simulink model "adaptiveControl_1DOF"  (R2021a)
settings: Solver=VariableStepAuto  StartTime=0.0  StopTime=50  RelTol=1e-3
values from neighbouring files (symbols this model uses):
  A = 0.2    [assignment8_main.m]
  Kd = 20    [assignment8_main.m]
  Khat_theta = 0.001    [assignment8_main.m]
  lambda = 10    [assignment8_main.m]
  omega = 0.5    [assignment8_main.m]
  theta_true = [myRobot_1DOF.I, myRobot_1DOF.F, myRobot_1DOF.G].'    [assignment8_main.m]
undefined symbols (not defined in the file or in its folder): myRobot_1DOF
settings Model: Creator=fabio  LastModifiedBy=fabio

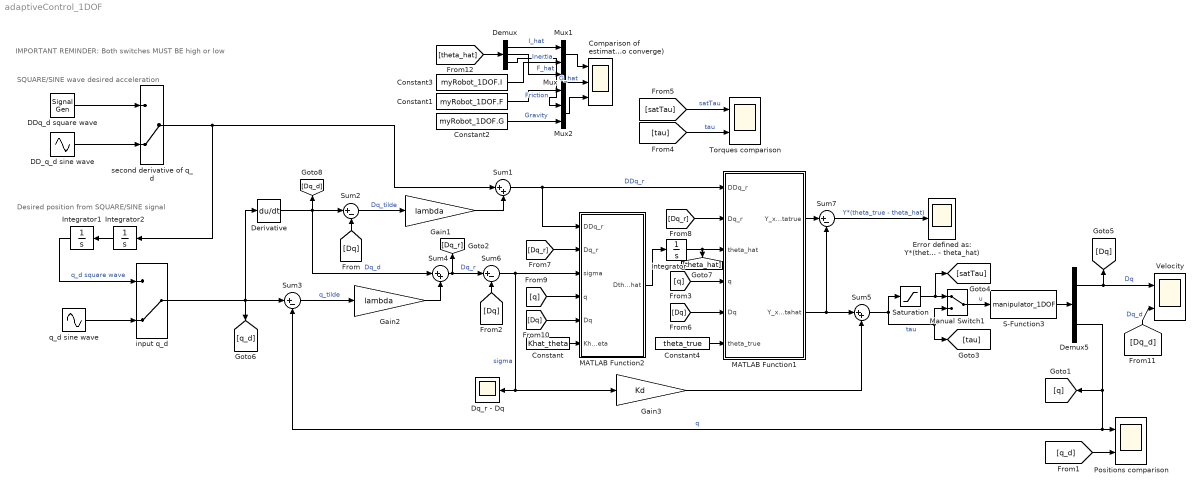
== system adaptiveControl_1DOF ==
  note: Desired position from SQUARE/SINE signal
  note: SQUARE/SINE wave desired acceleration
  note: IMPORTANT REMINDER: Both switches MUST BE high or low
  Comparison of estimated and real parameters (they don't necessarely have to converge) : Scope  NumInputPorts=3
  Constant : Constant  Value=Khat_theta  VectorParams1D=off
  Constant1 : Constant  Value=myRobot_1DOF.F
  Constant2 : Constant  Value=myRobot_1DOF.G
  Constant3 : Constant  Value=myRobot_1DOF.I  VectorParams1D=off
  Constant4 : Constant  Value=theta_true
  "DD_q_d sine wave " : Sin  Amplitude=-A*omega*omega  Frequency=omega  SampleTime=0
  DDq_d square wave : SignalGenerator  WaveForm=square  Amplitude=A  Frequency=omega*2  Units=rad/sec
  Demux : Demux  Outputs=3
  Demux5 : Demux  Outputs=[1 1]
  Derivative : Derivative
  Dq_r - Dq : Scope
  Error defined as: Y*(theta_true - theta_hat) : Scope
  Gain1 : Gain  Gain=lambda
  Gain2 : Gain  Gain=lambda
  Gain3 : Gain  Gain=Kd
  Integrator : Integrator  InitialCondition=myRobot_1DOF.theta_hat_0
  Integrator1 : Integrator
  Integrator2 : Integrator
  MATLAB Function1 : MATLAB Function  TreatAsAtomicUnit=on
  MATLAB Function2 : MATLAB Function  TreatAsAtomicUnit=on
  Manual Switch1 : ManualSwitch
  Mux : Mux  Inputs=2
  Mux1 : Mux  Inputs=2
  Mux2 : Mux  Inputs=2
  Positions comparison : Scope  NumInputPorts=2
  S-Function3 : S-Function  FunctionName=manipulator_1DOF  Parameters=myRobot_1DOF  SFunctionDeploymentMode=off  EnableBusSupport=off
  Saturation : Saturate  UpperLimit=20  LowerLimit=-20
  Sum1 : Sum  Inputs=|++
  Sum{2..3,6..7} (4 alike) : Sum  Inputs=|+-
  Sum4 : Sum  Inputs=|++
  Sum5 : Sum  Inputs=|++
  Torques comparison : Scope  NumInputPorts=2
  Velocity : Scope  NumInputPorts=2
  input q_d : ManualSwitch  CurrentSetting=0
  q_d sine wave : Sin  Amplitude=A  Frequency=omega  SampleTime=0
  second derivative of q_d : ManualSwitch  CurrentSetting=0
  wires:
  Manual Switch1/1 -> S-Function3/1  "u"
  Sum2/1 -> Gain1/1  "Dq_tilde"
  Saturation/1 -> Manual Switch1/1, [satTau]
  S-Function3/1 -> Demux5/1
  Demux5/1 -> [Dq], Velocity/1  "Dq"
  Demux5/2 -> Sum3/2, Positions comparison/1, [q]  "q"
  Sum3/1 -> Gain2/1  "q_tilde"
  Derivative/1 -> Sum4/1, Sum2/1, [Dq_d]  "Dq_d"
  Gain1/1 -> Sum1/2
  Gain2/1 -> Sum4/2
  Sum4/1 -> Sum6/1, [Dq_r]  "Dq_r"
  Sum1/1 -> MATLAB Function2/1(DDq_r), MATLAB Function1/1(DDq_r)  "DDq_r"
  [Dq] -> Sum6/2
  [Dq] -> Sum2/2
  Sum6/1 -> Dq_r - Dq/1, Gain3/1, MATLAB Function2/3(sigma)  "sigma"
  MATLAB Function2/1(Dtheta_hat) -> Integrator/1
  Integrator/1 -> [theta_hat], MATLAB Function1/3(theta_hat)
  Gain3/1 -> Sum5/2
  Sum5/1 -> Manual Switch1/2, [tau], Saturation/1  "tau"
  [q] -> MATLAB Function1/4(q)
  [Dq] -> MATLAB Function1/5(Dq)
  [Dq_r] -> MATLAB Function2/2(Dq_r)
  [Dq_r] -> MATLAB Function1/2(Dq_r)
  [q] -> MATLAB Function2/4(q)
  [Dq] -> MATLAB Function2/5(Dq)
  [q_d] -> Positions comparison/2
  Constant/1 -> MATLAB Function2/6(Khat_theta)
  [Dq_d] -> Velocity/2  "Dq_d"
  [satTau] -> Torques comparison/1  "satTau"
  [tau] -> Torques comparison/2  "tau"
  MATLAB Function1/2(Y_x_thetahat) -> Sum5/1, Sum7/2
  Sum7/1 -> Error defined as: Y*(theta_true - theta_hat)/1  "Y*(theta_true - theta_hat)"
  Constant4/1 -> MATLAB Function1/6(theta_true)
  MATLAB Function1/1(Y_x_thetatrue) -> Sum7/1
  q_d sine wave/1 -> input q_d/2
  DDq_d square wave/1 -> second derivative of q_d/1
  "DD_q_d sine wave "/1 -> second derivative of q_d/2
  second derivative of q_d/1 -> Integrator2/1, Sum1/1
  Integrator2/1 -> Integrator1/1
  Integrator1/1 -> input q_d/1  "q_d square wave"
  input q_d/1 -> Derivative/1, [q_d], Sum3/1
  Constant2/1 -> Mux2/2  "Gravity"
  Demux/2 -> Mux/1  "F_hat"
  Mux/1 -> Comparison of estimated and real parameters (they don't necessarely have to converge)/2
  Constant1/1 -> Mux/2  "Friction"
  Demux/3 -> Mux2/1  "G_hat"
  Constant3/1 -> Mux1/2  "Inertia"
  Mux2/1 -> Comparison of estimated and real parameters (they don't necessarely have to converge)/3
  Demux/1 -> Mux1/1  "I_hat"
  Mux1/1 -> Comparison of estimated and real parameters (they don't necessarely have to converge)/1
  [theta_hat] -> Demux/1

== matlab function adaptiveControl_1DOF/MATLAB Function1 ==
  data: Y_x_thetatrue output; DDq_r input; Dq_r input; theta_hat input; Y_x_thetahat output; q input; Dq input; theta_true input
function [Y_x_thetatrue, Y_x_thetahat] = Y(DDq_r, Dq_r, theta_hat, q, Dq, theta_true)

    Y = [DDq_r, Dq, sin(q)];
    Y_x_thetahat = Y * theta_hat;
    Y_x_thetatrue = Y * theta_true;
end

== matlab function adaptiveControl_1DOF/MATLAB Function2 ==
  data: DDq_r input; Dq_r input; sigma input; Dtheta_hat output; q input; Dq input; Khat_theta input
function Dtheta_hat = invK_x_Y(DDq_r, Dq_r, sigma, q, Dq, Khat_theta)

    Y = [DDq_r, Dq, sin(q)];

    Dtheta_hat = inv(Khat_theta) * Y.' * sigma;
end
